simulink model "NumSim_standard_eVTOL"  (R2024b)
settings: Solver=ode14x  StartTime=0.0  StopTime=250  FixedStep=0.005  RelTol=1e-3
values from neighbouring files (symbols this model uses):
  aDl =     [initdata.mat]
  aDr =     [initdata.mat]
  aDyn =     [initdata.mat]
  Airport = init_airport('PHNL')    [initdata_HIL_eVTOL.m]
  aLat =     [initdata.mat]
  aLon =     [initdata.mat]
  D = Prop.D    [EOM_dt_MC.m]    (also in EOM_get_alf_dt_de_prop_evtol.m = CD * QS)
  dt0 = X(2)    [EOM_get_alf_dt_de_prop_evtol.m]    (also in initdata.mat = 0.258252593971; initdata_HIL_eVTOL.m = EOM_dt_MC)
  EAS0 = TAS0 / EAS2TAS    [initdata_HIL_eVTOL.m]
  FCS = init_FCS    [initdata_HIL_eVTOL.m]
  General = init_layoutdata    [EOM_dt_MC.m]    (also in build_optimized_CA.m; initdata.mat = ; initdata_HIL_eVTOL.m)
  h0 = Con(1)    [EOM_get_alf_dt_de_prop_evtol.m]    (also in initdata.mat = 450; initdata_HIL_eVTOL.m = 50)
  mass = Con(3)    [EOM_get_alf_dt_de_prop_evtol.m]    (also in initdata.mat = 2255.54; initdata_HIL_eVTOL.m = 7)
  Motor = init_motor_evtol    [EOM_dt_MC.m]    (also in initdata.mat = []; initdata_HIL_eVTOL.m)
  Prop = init_propeller_evtol_new    [EOM_dt_MC.m]    (also in initdata_HIL_eVTOL.m)
  R2D = 180/pi    (= 57.2957795131)    [EOM_get_alf_dt_de_prop_evtol.m]    (also in init_FCS.m; init_aerodata_evtol.m; init_airport.m; initdata.mat)
  theta0 = -0.0510981441662    [initdata.mat]
undefined symbols (not defined in the file or in its folder): A1, aDa, aDe, asbhl20env, B1, C1, de0, Earth, Environment, InitData, Kd, Kp, magnitude, Tc, WGS84
libraries: simulink_extras x26, simulink x18, slpidlib x14, vrlib x8, matrix_library x6, sharedutil x6, sharedtransform x5, aerolibwindfilters x4, aerolibatmos2 x3, aerolibobsolete x2, aerolibactuator x2, aerolibasang x2
(part 6 of 7)

== system NumSim_standard_eVTOL/Environment/Wind Models/Dryden Wind Turbulence Model (Continuous (+q -r))/Select angular rates/Interpolate rates ==
  pgw_h&l : Inport
  qgw_h&l : Inport  Port=2
  rgw_h&l : Inport  Port=3
  DCM : Inport  Port=4
  Wind direction : Inport  Port=5
  Altitude : Inport  Port=6
  Action Port : ActionPort  PropagateVarSize=During execution  ActionPortLabel=else
  Mux : Mux  Inputs=3
  Mux1 : Mux  Inputs=3
  Product1 : Product  Inputs=**/  SaturateOnIntegerOverflow=on  OutDataTypeStr=Inherit: Same as first input
  Selector : Selector  InputPortWidth=2  IndexOptions=Index vector (dialog)  Indices=1  OutputSizes=1
  Selector1 : Selector  InputPortWidth=2  IndexOptions=Index vector (dialog)  Indices=1  OutputSizes=1
  Selector2 : Selector  InputPortWidth=2  IndexOptions=Index vector (dialog)  Indices=1  OutputSizes=1
  Selector3 : Selector  InputPortWidth=2  IndexOptions=Index vector (dialog)  Indices=2  OutputSizes=1
  Selector4 : Selector  InputPortWidth=2  IndexOptions=Index vector (dialog)  Indices=2  OutputSizes=1
  Selector5 : Selector  InputPortWidth=2  IndexOptions=Index vector (dialog)  Indices=2  OutputSizes=1
  Sum : Sum  Inputs=|-+  SaturateOnIntegerOverflow=on
  Sum1 : Sum  Inputs=|+-  SaturateOnIntegerOverflow=on
  Sum2 : Sum  Inputs=-+|  SaturateOnIntegerOverflow=on
  Sum3 : Sum  Inputs=++|  SaturateOnIntegerOverflow=on
  max_height_low : Constant  Value=max_height_low
  min_height_high : Constant  Value=min_height_high
  wind to body transformation : Subsystem
  pgw,qgw,rgw : Outport  InitialOutput=0  VectorParamsAs1DForOutWhenUnconnected=off
  wires:
  Mux/1 -> wind to body transformation/3(pg_l,qg_l,rg_l)
  DCM/1 -> wind to body transformation/1(DCM)
  wind to body transformation/1(pg,qg,rg) -> Sum3/1, Sum2/1
  Sum3/1 -> pgw,qgw,rgw/1
  Product1/1 -> Sum3/2
  Mux1/1 -> Sum2/2
  Sum2/1 -> Product1/1
  Sum1/1 -> Product1/2
  Sum/1 -> Product1/3
  Altitude/1 -> Sum1/1
  min_height_high/1 -> Sum/2
  max_height_low/1 -> Sum1/2, Sum/1
  Wind direction/1 -> wind to body transformation/2(Wind direction)
  Selector3/1 -> Mux1/1
  Selector4/1 -> Mux1/2
  Selector5/1 -> Mux1/3
  pgw_h&l/1 -> Selector/1, Selector3/1
  qgw_h&l/1 -> Selector4/1, Selector1/1
  rgw_h&l/1 -> Selector5/1, Selector2/1
  Selector/1 -> Mux/1
  Selector1/1 -> Mux/2
  Selector2/1 -> Mux/3

== system NumSim_standard_eVTOL/Environment/Wind Models/Dryden Wind Turbulence Model (Continuous (+q -r))/Select angular rates/Low altitude rates ==
  DCM : Inport
  pgw_h&l : Inport  Port=2
  qgw_h&l : Inport  Port=3
  rgw_h&l : Inport  Port=4
  Wind direction : Inport  Port=5
  Action Port : ActionPort  PropagateVarSize=During execution  ActionPortLabel=if(u1<=max_height_low)
  Mux : Mux  Inputs=3
  Selector : Selector  InputPortWidth=2  IndexOptions=Index vector (dialog)  Indices=1  OutputSizes=1
  Selector1 : Selector  InputPortWidth=2  IndexOptions=Index vector (dialog)  Indices=1  OutputSizes=1
  Selector2 : Selector  InputPortWidth=2  IndexOptions=Index vector (dialog)  Indices=1  OutputSizes=1
  wind to body transformation : Subsystem
  pgw,qgw,rgw : Outport  InitialOutput=0  VectorParamsAs1DForOutWhenUnconnected=off
  wires:
  DCM/1 -> wind to body transformation/1(DCM)
  pgw_h&l/1 -> Selector/1
  qgw_h&l/1 -> Selector1/1
  rgw_h&l/1 -> Selector2/1
  Selector/1 -> Mux/1
  Selector1/1 -> Mux/2
  Selector2/1 -> Mux/3
  Mux/1 -> wind to body transformation/3(pg_l,qg_l,rg_l)
  wind to body transformation/1(pg,qg,rg) -> pgw,qgw,rgw/1
  Wind direction/1 -> wind to body transformation/2(Wind direction)

== system NumSim_standard_eVTOL/Environment/Wind Models/Dryden Wind Turbulence Model (Continuous (+q -r))/Select angular rates/Medium//High altitude rates ==
  pgw_h&l : Inport
  qgw_h&l : Inport  Port=2
  rgw_h&l : Inport  Port=3
  Action Port : ActionPort  PropagateVarSize=During execution  ActionPortLabel=elseif(u1>=min_height_high)
  Gain : Gain  SaturateOnIntegerOverflow=on  OutDataTypeStr=Inherit: Same as input  ParamDataTypeStr=Inherit: Same as input
  Mux : Mux  Inputs=3
  Selector3 : Selector  InputPortWidth=6  IndexOptions=Index vector (dialog)  Indices=[ 2 4 6]  OutputSizes=1
  pgw,qgw,rgw : Outport  InitialOutput=0  VectorParamsAs1DForOutWhenUnconnected=off
  wires:
  Gain/1 -> pgw,qgw,rgw/1
  Selector3/1 -> Gain/1
  pgw_h&l/1 -> Mux/1
  qgw_h&l/1 -> Mux/2
  rgw_h&l/1 -> Mux/3
  Mux/1 -> Selector3/1

== system NumSim_standard_eVTOL/Environment/Wind Models/Dryden Wind Turbulence Model (Continuous (+q -r))/Select angular rates/Merge Subsystems ==
  low : Inport
  high : Inport  Port=2
  interpolated : Inport  Port=3
  Demux : Demux  Outputs=3
      settings: DisplayOption=none
  Merge : Merge  Inputs=3
  pgw : Outport  VectorParamsAs1DForOutWhenUnconnected=off
  qgw : Outport  Port=2  VectorParamsAs1DForOutWhenUnconnected=off
  rgw : Outport  Port=3  VectorParamsAs1DForOutWhenUnconnected=off
  wires:
  low/1 -> Merge/1
  high/1 -> Merge/2
  interpolated/1 -> Merge/3
  Demux/2 -> qgw/1
  Demux/3 -> rgw/1
  Demux/1 -> pgw/1
  Merge/1 -> Demux/1

== system NumSim_standard_eVTOL/Environment/Wind Models/Dryden Wind Turbulence Model (Continuous (+q -r))/Select velocities/Interpolate velocities ==
  ugw_h&l : Inport
  vgw_h&l : Inport  Port=2
  wgw_h&l : Inport  Port=3
  DCM : Inport  Port=4
  Wind direction : Inport  Port=5
  Altitude : Inport  Port=6
  Action Port : ActionPort  PropagateVarSize=During execution  ActionPortLabel=else
  Mux : Mux  Inputs=3
  Mux1 : Mux  Inputs=3
  Product1 : Product  Inputs=**/  SaturateOnIntegerOverflow=on  OutDataTypeStr=Inherit: Same as first input
  Selector : Selector  InputPortWidth=2  IndexOptions=Index vector (dialog)  Indices=1  OutputSizes=1
  Selector1 : Selector  InputPortWidth=2  IndexOptions=Index vector (dialog)  Indices=1  OutputSizes=1
  Selector2 : Selector  InputPortWidth=2  IndexOptions=Index vector (dialog)  Indices=1  OutputSizes=1
  Selector3 : Selector  InputPortWidth=2  IndexOptions=Index vector (dialog)  Indices=2  OutputSizes=1
  Selector4 : Selector  InputPortWidth=2  IndexOptions=Index vector (dialog)  Indices=2  OutputSizes=1
  Selector5 : Selector  InputPortWidth=2  IndexOptions=Index vector (dialog)  Indices=2  OutputSizes=1
  Sum : Sum  Inputs=|-+  SaturateOnIntegerOverflow=on
  Sum1 : Sum  Inputs=|+-  SaturateOnIntegerOverflow=on
  Sum2 : Sum  Inputs=-+|  SaturateOnIntegerOverflow=on
  Sum3 : Sum  Inputs=++|  SaturateOnIntegerOverflow=on
  max_height_low : Constant  Value=max_height_low
  min_height_high : Constant  Value=min_height_high
  wind to body transformation : Subsystem
  ugw,vgw,wgw : Outport  InitialOutput=0  VectorParamsAs1DForOutWhenUnconnected=off
  wires:
  Mux/1 -> wind to body transformation/3(ug_l,vg_l,wg_l)
  Wind direction/1 -> wind to body transformation/2(Wind direction)
  DCM/1 -> wind to body transformation/1(DCM)
  wind to body transformation/1(ug,vg,wg) -> Sum3/1, Sum2/1
  Sum3/1 -> ugw,vgw,wgw/1
  Product1/1 -> Sum3/2
  Mux1/1 -> Sum2/2
  Sum2/1 -> Product1/1
  Sum1/1 -> Product1/2
  Sum/1 -> Product1/3
  Altitude/1 -> Sum1/1
  min_height_high/1 -> Sum/2
  max_height_low/1 -> Sum1/2, Sum/1
  Selector3/1 -> Mux1/1
  Selector4/1 -> Mux1/2
  Selector5/1 -> Mux1/3
  ugw_h&l/1 -> Selector/1, Selector3/1
  vgw_h&l/1 -> Selector4/1, Selector1/1
  wgw_h&l/1 -> Selector5/1, Selector2/1
  Selector/1 -> Mux/1
  Selector1/1 -> Mux/2
  Selector2/1 -> Mux/3

== system NumSim_standard_eVTOL/Environment/Wind Models/Dryden Wind Turbulence Model (Continuous (+q -r))/Select velocities/Low altitude velocities ==
  DCM : Inport
  ugw_h&l : Inport  Port=2
  vgw_h&l : Inport  Port=3
  wgw_h&l : Inport  Port=4
  Wind direction : Inport  Port=5
  Action Port : ActionPort  PropagateVarSize=During execution  ActionPortLabel=if(u1<=max_height_low)
  Mux : Mux  Inputs=3
  Selector : Selector  InputPortWidth=2  IndexOptions=Index vector (dialog)  Indices=1  OutputSizes=1
  Selector1 : Selector  InputPortWidth=2  IndexOptions=Index vector (dialog)  Indices=1  OutputSizes=1
  Selector2 : Selector  InputPortWidth=2  IndexOptions=Index vector (dialog)  Indices=1  OutputSizes=1
  wind to body transformation : Subsystem
  ugw,vgw,wgw : Outport  InitialOutput=0  VectorParamsAs1DForOutWhenUnconnected=off
  wires:
  Mux/1 -> wind to body transformation/3(ug_l,vg_l,wg_l)
  Selector2/1 -> Mux/3
  wind to body transformation/1(ug,vg,wg) -> ugw,vgw,wgw/1
  Wind direction/1 -> wind to body transformation/2(Wind direction)
  DCM/1 -> wind to body transformation/1(DCM)
  Selector1/1 -> Mux/2
  Selector/1 -> Mux/1
  wgw_h&l/1 -> Selector2/1
  vgw_h&l/1 -> Selector1/1
  ugw_h&l/1 -> Selector/1

== system NumSim_standard_eVTOL/Environment/Wind Models/Dryden Wind Turbulence Model (Continuous (+q -r))/Select velocities/Medium//High altitude velocities ==
  ugw_h&l : Inport
  vgw_h&l : Inport  Port=2
  wgw_h&l : Inport  Port=3
  Action Port : ActionPort  PropagateVarSize=During execution  ActionPortLabel=elseif(u1>=min_height_high)
  Gain : Gain  SaturateOnIntegerOverflow=on  OutDataTypeStr=Inherit: Same as input  ParamDataTypeStr=Inherit: Same as input
  Mux : Mux  Inputs=3
  Selector3 : Selector  InputPortWidth=6  IndexOptions=Index vector (dialog)  Indices=[ 2 4 6]  OutputSizes=1
  ugw,vgw,wgw : Outport  InitialOutput=0  VectorParamsAs1DForOutWhenUnconnected=off
  wires:
  vgw_h&l/1 -> Mux/2
  Gain/1 -> ugw,vgw,wgw/1
  Selector3/1 -> Gain/1
  Mux/1 -> Selector3/1
  wgw_h&l/1 -> Mux/3
  ugw_h&l/1 -> Mux/1

== system NumSim_standard_eVTOL/Environment/Wind Models/Dryden Wind Turbulence Model (Continuous (+q -r))/Select velocities/Merge Subsystems ==
  low : Inport
  high : Inport  Port=2
  interpolated : Inport  Port=3
  Demux : Demux  Outputs=3
      settings: DisplayOption=none
  Merge : Merge  Inputs=3
  ugw : Outport  VectorParamsAs1DForOutWhenUnconnected=off
  vgw : Outport  Port=2  VectorParamsAs1DForOutWhenUnconnected=off
  wgw : Outport  Port=3  VectorParamsAs1DForOutWhenUnconnected=off
  wires:
  Merge/1 -> Demux/1
  Demux/1 -> ugw/1
  Demux/3 -> wgw/1
  Demux/2 -> vgw/1
  interpolated/1 -> Merge/3
  high/1 -> Merge/2
  low/1 -> Merge/1

== system NumSim_standard_eVTOL/Environment/Wind Models/Dryden Wind Turbulence Model (Continuous (+q -r))/Turbulence scale lengths/Low altitude scale length ==
  h : Inport
  Limit Function 10ft to 1000ft : Saturate  UpperLimit=max_height_low  LowerLimit=10
  Low Altitude Scale Length : Fcn  Expr=u(1)/(0.177+0.000823*u(1))^1.2
  L_ug L_vg : Outport  InitialOutput=0  VectorParamsAs1DForOutWhenUnconnected=off
  L_wg : Outport  Port=2  InitialOutput=0  VectorParamsAs1DForOutWhenUnconnected=off
  wires:
  h/1 -> Limit Function 10ft to 1000ft/1
  Low Altitude Scale Length/1 -> L_ug L_vg/1
  Limit Function 10ft to 1000ft/1 -> L_wg/1, Low Altitude Scale Length/1

== system NumSim_standard_eVTOL/Environment/Wind Models/Dryden Wind Turbulence Model (Continuous (+q -r))/Turbulence scale lengths/Medium//High altitude scale length ==
  Length Conversion : Subsystem
  Medium/High Altitude : Constant  Value=L_high
  L_ug L_vg L_wg : Outport  Unit=ft  InitialOutput=0  VectorParamsAs1DForOutWhenUnconnected=off
  wires:
  Medium/High Altitude/1 -> Length Conversion/1(in)
  Length Conversion/1(out) -> L_ug L_vg L_wg/1

== system NumSim_standard_eVTOL/FCS/FW/TECS/TECS PX4 & AP201/1st order filter2 ==
  In1 : Inport
  Delay : Delay  DelayLength=1
  Gain : Gain  Gain=0.05
  Gain1 : Gain  Gain=0.95
  Sum : Sum  Inputs=|++
  Out1 : Outport  VectorParamsAs1DForOutWhenUnconnected=off
  wires:
  Sum/1 -> Gain1/1, Out1/1
  Gain/1 -> Sum/1
  Delay/1 -> Sum/2
  Gain1/1 -> Delay/1
  In1/1 -> Gain/1

== system NumSim_standard_eVTOL/FCS/FW/TECS/TECS PX4 & AP201/thetac_AP201 ==
  LonMod : Inport
  SPE_RATE_C : Inport  Port=2
  SKE_RATE_C : Inport  Port=3
  SPE_RATE : Inport  Port=4
  SKE_RATE : Inport  Port=5
  Add15 : Sum  Inputs=+-|
  Add18 : Sum  Inputs=+-|
  Add20 : Sum  Inputs=+-|
  Add3 : Sum  Inputs=++|
  Detect Change : simulink/Logic and Bit Operations/Detect Change  vinit=0  OutDataTypeStr=boolean
  Divide{5..6,11..12} (4 alike) : Product  Inputs=**
  Divide7 : Product  Inputs=*/
  Integrator : Integrator  ExternalReset=either  LimitOutput=on  UpperSaturationLimit=FCS.theta_max*0.6  LowerSaturationLimit=FCS.theta_min*0.6  ZeroCross=off
  KEI : Gain  Gain=0.2
  "KEP " : Gain  Gain=0.2
  Radians to Degrees : simulink_extras/Transformations/Radians to Degrees
  Saturation Dynamic2 : simulink/Discontinuities/Saturation Dynamic  OutMin=[]  OutMax=[]  OutDataTypeStr=Inherit: Same as second input  OutDataType=fixdt(1, 16)  OutScaling=2^-10  DoSatur=off
  dD_dot scp : Scope
  g1 : Gain  Gain=9.8
  thetac scp1 : Scope
  thetac_AP1 : Scope  NumInputPorts=2
  thetac_AP201 : Scope  NumInputPorts=2
  thetac : Outport  VectorParamsAs1DForOutWhenUnconnected=off
  wires:
  [V] -> g1/1
  g1/1 -> Divide7/2
  Divide7/1 -> KEI/1, "KEP "/1, dD_dot scp/1  "dD_dot"
  KEI/1 -> Integrator/1
  SPE_RATE_C/1 -> Divide5/1
  [theta_min] -> Saturation Dynamic2/3
  Divide12/1 -> Add18/2
  [SPE_wt] -> Divide11/2, Divide5/2  "SPE_WT"
  [SKE_wt] -> Divide12/2, Divide6/2  "SKE_WT"
  Add20/1 -> Divide7/1  "SEB_rate_err"
  SKE_RATE/1 -> Divide12/1
  Integrator/1 -> Add3/1, thetac_AP201/1
  [theta_max] -> Saturation Dynamic2/1
  SKE_RATE_C/1 -> Divide6/1
  Divide5/1 -> Add15/1
  Divide6/1 -> Add15/2
  Add15/1 -> Add20/1  "SEB_rate_c"
  SPE_RATE/1 -> Divide11/1
  Add18/1 -> Add20/2  "SEB_rate"
  Divide11/1 -> Add18/1
  "KEP "/1 -> thetac_AP201/2, Add3/2
  Saturation Dynamic2/1 -> Radians to Degrees/1, thetac/1
  Add3/1 -> Saturation Dynamic2/2
  LonMod/1 -> thetac_AP1/1, Detect Change/1
  Detect Change/1 -> thetac_AP1/2, Integrator/2
  Radians to Degrees/1 -> thetac scp1/1

== system NumSim_standard_eVTOL/FCS/FW/TECS/TECS PX4 & AP201/throttlec_AP201 ==
  LonMod : Inport
  SPE_RATE_C : Inport  Port=2
  SKE_RATE_C : Inport  Port=3
  SPE_RATE : Inport  Port=4
  SKE_RATE : Inport  Port=5
  Add2 : Sum  Inputs=++|
  Add6 : Sum  Inputs=++|
  Add7 : Sum  Inputs=++|
  Add9 : Sum  Inputs=+-|
  Detect Change : simulink/Logic and Bit Operations/Detect Change  vinit=0  OutDataTypeStr=boolean
  Divide2 : Product  Inputs=*/
  Integrator1 : Integrator  ExternalReset=either  LimitOutput=on  UpperSaturationLimit=0.5  LowerSaturationLimit=-0.5  ZeroCross=off
  KTI : Gain  Gain=0.8
  KTP : Gain  Gain=0.4
  PX4 1st order filter (time depended)1 : CustomLib/PX4 1st order filter (time depended)  Commented=on  Ts=0.2
  Rate Limiter Dynamic1 : simulink/Discontinuities/Rate Limiter Dynamic
  Saturation Dynamic : simulink/Discontinuities/Saturation Dynamic  OutMin=[]  OutMax=[]  OutDataTypeStr=Inherit: Same as second input  OutDataType=fixdt(1, 16)  OutScaling=2^-10  DoSatur=off
  Saturation3 : Saturate  UpperLimit=1  LowerLimit=-1
  dE_dot scp : Scope
  dt scp{2..5} (4 alike) : Scope
  dt_slew : Constant  Value=0.8
  dti scp1 : Scope  NumInputPorts=2
  g12 : Gain  Gain=9.8
  g13 : Gain  Gain=-1
  dt : Outport  VectorParamsAs1DForOutWhenUnconnected=off
  wires:
  Add2/1 -> Rate Limiter Dynamic1/2  "dt"
  Saturation Dynamic/1 -> dt scp4/1, Add9/1  "STE_rate_c"
  Rate Limiter Dynamic1/1 -> Saturation3/1
  [STE_rate_min] -> Saturation Dynamic/3
  Add7/1 -> dt scp5/1, Saturation Dynamic/2  "STE_rate_c"
  Divide2/1 -> dE_dot scp/1, KTI/1, KTP/1  "dE_dot"
  g12/1 -> Divide2/2
  SPE_RATE/1 -> Add6/1
  Add9/1 -> Divide2/1  "STE_rate_err"
  [V] -> g12/1
  KTI/1 -> Integrator1/1
  SKE_RATE/1 -> Add6/2
  KTP/1 -> Add2/2, dti scp1/2
  Add6/1 -> dt scp3/1, Add9/2  "STE_rate"
  SKE_RATE_C/1 -> Add7/2
  SPE_RATE_C/1 -> Add7/1
  [STE_rate_max] -> Saturation Dynamic/1
  Integrator1/1 -> Add2/1, dti scp1/1
  dt_slew/1 -> Rate Limiter Dynamic1/1, g13/1
  g13/1 -> Rate Limiter Dynamic1/3
  Saturation3/1 -> dt/1, dt scp2/1
  LonMod/1 -> Detect Change/1
  Detect Change/1 -> Integrator1/2

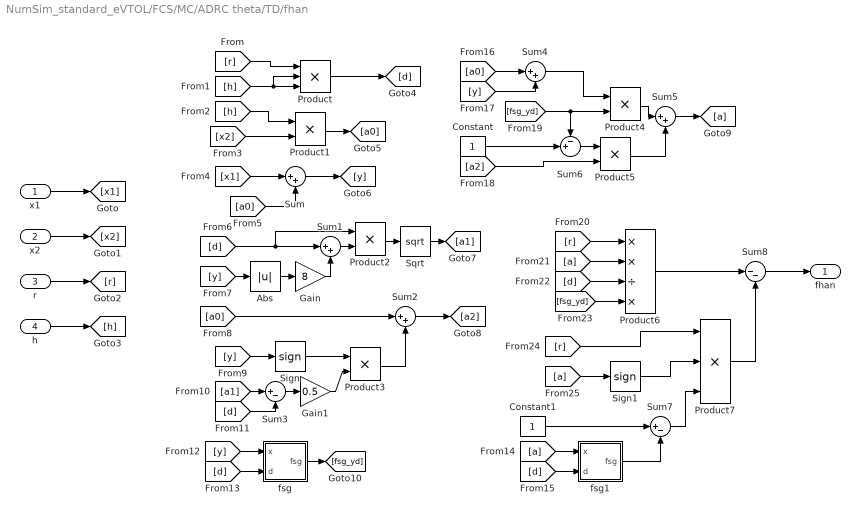
== system NumSim_standard_eVTOL/FCS/MC/ADRC theta/TD/fhan ==
  x1 : Inport
  x2 : Inport  Port=2
  r : Inport  Port=3
  h : Inport  Port=4
  Abs : Abs  SaturateOnIntegerOverflow=off
  Constant : Constant
  Constant1 : Constant
  Gain : Gain  Gain=8
  Gain1 : Gain  Gain=0.5
  Product : Product  Inputs=3
  Product{1..5} (5 alike) : Product
  Product6 : Product  Inputs=**/*
  Product7 : Product  Inputs=***
  Sign : Signum
  Sign1 : Signum
  Sqrt : Sqrt
  Sum{,1..2,4..5} (5 alike) : Sum  Inputs=|++
  Sum3 : Sum  Inputs=|+-
  Sum6 : Sum  Inputs=-+|
  Sum7 : Sum  Inputs=|+-
  Sum8 : Sum  Inputs=|--
  fsg : Subsystem
  fsg1 : Subsystem
  fhan : Outport
  wires:
  Product/1 -> [d]
  x1/1 -> [x1]
  x2/1 -> [x2]
  r/1 -> [r]
  h/1 -> [h]
  [r] -> Product/1
  [h] -> Product/3, Product/2
  [h] -> Product1/1
  [x2] -> Product1/2
  Product1/1 -> [a0]
  [x1] -> Sum/1
  [a0] -> Sum/2
  Sum/1 -> [y]
  [d] -> Sum1/1, Product2/1
  [y] -> Abs/1
  Abs/1 -> Gain/1
  Gain/1 -> Sum1/2
  Sum1/1 -> Product2/2
  Product2/1 -> Sqrt/1
  [a0] -> Sum2/1
  [y] -> Sign/1
  Sign/1 -> Product3/1
  [a1] -> Sum3/1
  [d] -> Sum3/2
  Sum3/1 -> Gain1/1
  Gain1/1 -> Product3/2
  Product3/1 -> Sum2/2
  Sum2/1 -> [a2]
  [y] -> fsg/1(x)
  [d] -> fsg/2(d)
  [d] -> fsg1/2(d)
  [a] -> fsg1/1(x)
  [a0] -> Sum4/1
  [y] -> Sum4/2
  Sum4/1 -> Product4/1
  Product4/1 -> Sum5/1
  [a2] -> Product5/2
  Constant/1 -> Sum6/2
  Sum6/1 -> Product5/1
  Product5/1 -> Sum5/2
  Sum5/1 -> [a]
  fsg/1(fsg) -> [fsg_yd]
  [fsg_yd] -> Sum6/1, Product4/2
  [r] -> Product6/1
  [a] -> Product6/2
  [d] -> Product6/3
  [fsg_yd] -> Product6/4
  Constant1/1 -> Sum7/1
  fsg1/1(fsg) -> Sum7/2
  [a] -> Sign1/1
  [r] -> Product7/1
  Sign1/1 -> Product7/2
  Sum7/1 -> Product7/3
  Product6/1 -> Sum8/1
  Product7/1 -> Sum8/2
  Sum8/1 -> fhan/1
  Sqrt/1 -> [a1]

== system NumSim_standard_eVTOL/airframe/force moment/aero F&M in body axis/Aerodynamic Coefficients/Actuator Increments ==
  Actuators : Inport
  incid : Inport  Port=2
  Aileron : Subsystem
  Bus Selector1 : BusSelector  OutputSignals=dl,dr,da
  Demux : Demux  Outputs=2
  Sum : Sum  Inputs=+++
  Terminator : Terminator
  V_left : Subsystem
  V_right : Subsystem
  cl : Outport  InitialOutput=0  VectorParamsAs1DForOutWhenUnconnected=off
  wires:
  Actuators/1 -> Bus Selector1/1
  Sum/1 -> cl/1
  V_right/1(dr_Coeff) -> Sum/2
  V_left/1(dl_Coeff) -> Sum/1
  Bus Selector1/1 -> V_left/2(dl)  "<dl>"
  Bus Selector1/3 -> Aileron/2(da)  "<da>"
  incid/1 -> Demux/1
  Demux/1 -> Aileron/1(alpha), V_right/1(alpha), V_left/1(alpha)  "alpha"
  Demux/2 -> Terminator/1  "beta"
  Aileron/1(da_Coeff) -> Sum/3
  Bus Selector1/2 -> V_right/2(dr)  "<dr>"

== system NumSim_standard_eVTOL/airframe/force moment/aero F&M in body axis/Aerodynamic Coefficients/Basic Coefficients ==
  Incid : Inport
  mach : Inport  Port=2
  2-D Lookup Table : Lookup_n-D  NumberOfTableDimensions=1  BreakpointsForDimension1=aLon.alpha  BreakpointsForDimension2=aLon.mach  BreakpointsForDimension3=aLon.flap  Table=aLon.CL  InternalRulePriority=Speed  RndMeth=Simplest
  2-D Lookup Table1 : Lookup_n-D  NumberOfTableDimensions=1  BreakpointsForDimension1=aLon.alpha  BreakpointsForDimension2=aLon.mach  BreakpointsForDimension3=aLon.flap  Table=aLon.CD  InternalRulePriority=Speed  RndMeth=Simplest
  2-D Lookup Table2 : Lookup_n-D  NumberOfTableDimensions=1  BreakpointsForDimension1=aLon.alpha  BreakpointsForDimension2=aLon.mach  BreakpointsForDimension3=aLon.flap  Table=aLon.Cm  InternalRulePriority=Speed  RndMeth=Simplest
  2-D Lookup Table3 : Lookup_n-D  BreakpointsForDimension1=aLat.beta  BreakpointsForDimension2=aLat.alpha  BreakpointsForDimension3=aLat.mach  Table=aLat.dCD  InternalRulePriority=Speed  RndMeth=Simplest
      settings: InputPortMap=u0,u1
  2-D Lookup Table4 : Lookup_n-D  BreakpointsForDimension1=aLat.beta  BreakpointsForDimension2=aLat.alpha  BreakpointsForDimension3=aLat.mach  Table=aLat.dCY  InternalRulePriority=Speed  RndMeth=Simplest
      settings: InputPortMap=u0,u1
  2-D Lookup Table5 : Lookup_n-D  BreakpointsForDimension1=aLat.beta  BreakpointsForDimension2=aLat.alpha  BreakpointsForDimension3=aLat.mach  Table=aLat.dCl  InternalRulePriority=Speed  RndMeth=Simplest
      settings: InputPortMap=u0,u1
  2-D Lookup Table6 : Lookup_n-D  BreakpointsForDimension1=aLat.beta  BreakpointsForDimension2=aLat.alpha  BreakpointsForDimension3=aLat.mach  Table=aLat.dCL  InternalRulePriority=Speed  RndMeth=Simplest
      settings: InputPortMap=u0,u1
  2-D Lookup Table7 : Lookup_n-D  BreakpointsForDimension1=aLat.beta  BreakpointsForDimension2=aLat.alpha  BreakpointsForDimension3=aLat.mach  Table=aLat.dCm  InternalRulePriority=Speed  RndMeth=Simplest
      settings: InputPortMap=u0,u1
  2-D Lookup Table8 : Lookup_n-D  BreakpointsForDimension1=aLat.beta  BreakpointsForDimension2=aLat.alpha  BreakpointsForDimension3=aLat.mach  Table=aLat.dCn  InternalRulePriority=Speed  RndMeth=Simplest
      settings: InputPortMap=u0,u1
  Constant : Constant  Value=0
  Constant1 : Constant  Value=0
  Demux : Demux  Outputs=2
  Display : Display
  Display1 : Display
  Gain : Gain
  Mux1 : Mux  Inputs=6
  Mux2 : Mux  Inputs=6
  Saturation : Saturate  UpperLimit=0.1  LowerLimit=0
  Scope{1..5} (5 alike) : Scope
  Sum5 : Sum  Inputs=+++  InputSameDT=on  SaturateOnIntegerOverflow=on  OutDataTypeStr=Inherit: Same as first input
  cl : Outport  InitialOutput=0  VectorParamsAs1DForOutWhenUnconnected=off
  wires:
  Mux1/1 -> Display/1, Sum5/2
  Demux/1 -> Scope5/1, [alpha]  "alpha"
  Demux/2 -> [beta]  "beta"
  2-D Lookup Table1/1 -> Mux1/2, Scope3/1  "CD"
  Constant1/1 -> Mux1/6, Mux1/4, Mux1/3
  2-D Lookup Table4/1 -> Mux2/3  "dCY"
  2-D Lookup Table5/1 -> Mux2/4  "dCl"
  2-D Lookup Table8/1 -> Mux2/6  "dCn"
  Sum5/1 -> cl/1
  Mux2/1 -> Sum5/3, Display1/1
  Incid/1 -> Demux/1
  [alpha] -> 2-D Lookup Table/1, Scope4/1
  2-D Lookup Table/1 -> Scope2/1, Mux1/1  "CL"
  [alpha] -> 2-D Lookup Table1/1
  [alpha] -> 2-D Lookup Table2/1
  2-D Lookup Table2/1 -> Gain/1  "Cm"
  [beta] -> 2-D Lookup Table6/1
  2-D Lookup Table6/1 -> Mux2/1  "dCL"
  [alpha] -> 2-D Lookup Table6/2
  [alpha] -> 2-D Lookup Table3/2
  [beta] -> 2-D Lookup Table3/1
  2-D Lookup Table3/1 -> Mux2/2  "dCD"
  [beta] -> 2-D Lookup Table4/1
  [alpha] -> 2-D Lookup Table4/2
  [alpha] -> 2-D Lookup Table5/2
  [beta] -> 2-D Lookup Table5/1
  [beta] -> 2-D Lookup Table7/1
  [alpha] -> 2-D Lookup Table7/2
  2-D Lookup Table7/1 -> Mux2/5  "dCm"
  [alpha] -> 2-D Lookup Table8/2
  [beta] -> 2-D Lookup Table8/1
  Constant/1 -> Sum5/1
  Saturation/1 -> Scope1/1, [mach]
  mach/1 -> Saturation/1
  Gain/1 -> Mux1/5

== system NumSim_standard_eVTOL/airframe/force moment/aero F&M in body axis/Aerodynamic Coefficients/Body Rate Damping ==
  Incid : Inport
  pqrn : Inport  Port=2
  alphaDot_n : Inport  Port=3
  1-D Lookup Table : Lookup_n-D  NumberOfTableDimensions=1  BreakpointsForDimension1=aDyn.alpha  BreakpointsForDimension2=aDyn.flap  Table=aDyn.CYp  InternalRulePriority=Speed  RndMeth=Simplest
  1-D Lookup Table1 : Lookup_n-D  NumberOfTableDimensions=1  BreakpointsForDimension1=aDyn.alpha  BreakpointsForDimension2=aDyn.flap  Table=aDyn.Clp  InternalRulePriority=Speed  RndMeth=Simplest
  1-D Lookup Table2 : Lookup_n-D  NumberOfTableDimensions=1  BreakpointsForDimension1=aDyn.alpha  BreakpointsForDimension2=aDyn.flap  Table=aDyn.Cnp  InternalRulePriority=Speed  RndMeth=Simplest
  1-D Lookup Table3 : Lookup_n-D  NumberOfTableDimensions=1  BreakpointsForDimension1=aDyn.alpha  BreakpointsForDimension2=aDyn.flap  Table=aDyn.CYr  InternalRulePriority=Speed  RndMeth=Simplest
  1-D Lookup Table4 : Lookup_n-D  NumberOfTableDimensions=1  BreakpointsForDimension1=aDyn.alpha  BreakpointsForDimension2=aDyn.flap  Table=aDyn.Clr  InternalRulePriority=Speed  RndMeth=Simplest
  1-D Lookup Table5 : Lookup_n-D  NumberOfTableDimensions=1  BreakpointsForDimension1=aDyn.alpha  BreakpointsForDimension2=aDyn.flap  Table=aDyn.Cnr  InternalRulePriority=Speed  RndMeth=Simplest
  1-D Lookup Table6 : Lookup_n-D  NumberOfTableDimensions=1  BreakpointsForDimension1=aDyn.alpha  BreakpointsForDimension2=aDyn.flap  Table=aDyn.CLq  InternalRulePriority=Speed  RndMeth=Simplest
  1-D Lookup Table7 : Lookup_n-D  NumberOfTableDimensions=1  BreakpointsForDimension1=aDyn.alpha  BreakpointsForDimension2=aDyn.flap  Table=aDyn.Cmq  InternalRulePriority=Speed  RndMeth=Simplest
  1-D Lookup Table8 : Lookup_n-D  NumberOfTableDimensions=1  BreakpointsForDimension1=aDyn.alpha  BreakpointsForDimension2=aDyn.flap  Table=aDyn.CLAlphaDot  InternalRulePriority=Speed  RndMeth=Simplest
  1-D Lookup Table9 : Lookup_n-D  NumberOfTableDimensions=1  BreakpointsForDimension1=aDyn.alpha  BreakpointsForDimension2=aDyn.flap  Table=aDyn.CmAlphaDot  InternalRulePriority=Speed  RndMeth=Simplest
  Add : Sum  Inputs=++++
  Constant{,6..7,13} (4 alike) : Constant  Value=0
  Demux : Demux  Outputs=3
  Demux1 : Demux  Outputs=2
  Mux{1..4} (4 alike) : Mux  Inputs=6
  Product{4..7} (4 alike) : Product  InputSameDT=on  SaturateOnIntegerOverflow=on  OutDataTypeStr=Inherit: Same as first input
  Terminator : Terminator
  cl : Outport  InitialOutput=0  VectorParamsAs1DForOutWhenUnconnected=off
  wires:
  Add/1 -> cl/1
  1-D Lookup Table/1 -> Mux1/3  "CYp"
  1-D Lookup Table2/1 -> Mux1/6  "Cnp"
  Mux1/1 -> Product4/1
  1-D Lookup Table1/1 -> Mux1/4  "Clp"
  pqrn/1 -> Demux/1
  Demux/1 -> [p]
  Demux/2 -> [q]
  Demux/3 -> [r]
  Constant/1 -> Mux1/1, Mux1/2, Mux1/5
  1-D Lookup Table7/1 -> Mux2/5  "Cmq"
  1-D Lookup Table6/1 -> Mux2/1  "CLq"
  Mux2/1 -> Product5/1
  1-D Lookup Table3/1 -> Mux3/3  "CYr"
  Mux3/1 -> Product6/1
  1-D Lookup Table4/1 -> Mux3/4  "Clr"
  1-D Lookup Table5/1 -> Mux3/6  "Cnr"
  Constant7/1 -> Mux3/2, Mux3/5, Mux3/1
  Constant13/1 -> Mux4/6, Mux4/4, Mux4/3, Mux4/2
  1-D Lookup Table9/1 -> Mux4/5  "CmAlphaDot"
  1-D Lookup Table8/1 -> Mux4/1  "CLAlphaDot"
  Constant6/1 -> Mux2/4, Mux2/6, Mux2/3, Mux2/2
  [p] -> Product4/2
  [q] -> Product5/2
  [r] -> Product6/2
  Mux4/1 -> Product7/1
  alphaDot_n/1 -> Product7/2
  Product4/1 -> Add/1
  Product7/1 -> Add/4
  Demux1/2 -> Terminator/1  "beta"
  Demux1/1 -> [alpha]  "alpha"
  Incid/1 -> Demux1/1
  Product5/1 -> Add/3
  [alpha] -> 1-D Lookup Table3/1, 1-D Lookup Table4/1, 1-D Lookup Table9/1, 1-D Lookup Table8/1, 1-D Lookup Table7/1, 1-D Lookup Table6/1, 1-D Lookup Table5/1, 1-D Lookup Table2/1, 1-D Lookup Table1/1, 1-D Lookup Table/1
  Product6/1 -> Add/2

== system NumSim_standard_eVTOL/airframe/force moment/aero F&M in body axis/Aerodynamic Coefficients/CLCDCY-CXCYCZ ==
  Incid : Inport
  Cl_LDY : Inport  Port=2
  Cl_xA : Fcn  Expr=-u[4]*cos(u[2])*cos(u[1])+u[3]*sin(u[1])
  Cl_yA : Fcn  Expr=-u[4]*sin(u[2])+u[5]
  Cl_zA : Fcn  Expr=-u[4]*cos(u[2])*sin(u[1])-u[3]*cos(u[1])
  Mux : Mux  Inputs=3
  Mux1 : Mux  Inputs=2
  Cl_XYZ : Outport  VectorParamsAs1DForOutWhenUnconnected=off
  wires:
  Mux/1 -> Cl_XYZ/1
  Cl_LDY/1 -> Mux1/2
  Incid/1 -> Mux1/1
  Cl_zA/1 -> Mux/3
  Cl_yA/1 -> Mux/2
  Cl_xA/1 -> Mux/1
  Mux1/1 -> Cl_zA/1, Cl_yA/1, Cl_xA/1

== system NumSim_standard_eVTOL/Environment/Wind Models/Dryden Wind Turbulence Model (Continuous (+q -r))/Select angular rates/Interpolate rates/wind to body transformation ==
  DCM : Inport
  Wind direction : Inport  Port=2
  pg_l,qg_l,rg_l : Inport  Port=3
  Demux : Demux  Outputs=3
      settings: DisplayOption=none
  Product : Product  Multiplication=Matrix(*)  SaturateOnIntegerOverflow=on  OutDataTypeStr=Inherit: Same as first input
  Reshape : Reshape  OutputDimensionality=Customize  OutputDimensions=[3,1]
  Reshape1 : Reshape
  Vector Concatenate : Concatenate  NumInputs=3
  convert to earth coords : Subsystem
  pg,qg,rg : Outport  VectorParamsAs1DForOutWhenUnconnected=off
  wires:
  Reshape1/1 -> pg,qg,rg/1
  Reshape/1 -> Product/2
  DCM/1 -> Product/1
  Wind direction/1 -> convert to earth coords/1(Wind direction)
  convert to earth coords/1(pg) -> Vector Concatenate/1
  convert to earth coords/2(qg) -> Vector Concatenate/2
  Vector Concatenate/1 -> Reshape/1
  Demux/1 -> convert to earth coords/2(pg_l)
  Demux/2 -> convert to earth coords/3(qg_l)
  Demux/3 -> Vector Concatenate/3
  Product/1 -> Reshape1/1
  pg_l,qg_l,rg_l/1 -> Demux/1

== system NumSim_standard_eVTOL/Environment/Wind Models/Dryden Wind Turbulence Model (Continuous (+q -r))/Select angular rates/Low altitude rates/wind to body transformation ==
  DCM : Inport
  Wind direction : Inport  Port=2
  pg_l,qg_l,rg_l : Inport  Port=3
  Demux : Demux  Outputs=3
      settings: DisplayOption=none
  Product : Product  Multiplication=Matrix(*)  SaturateOnIntegerOverflow=on  OutDataTypeStr=Inherit: Same as first input
  Reshape : Reshape  OutputDimensionality=Column vector (2-D)
  Reshape1 : Reshape
  Vector Concatenate : Concatenate  NumInputs=3
  convert to earth coords : Subsystem
  pg,qg,rg : Outport  VectorParamsAs1DForOutWhenUnconnected=off
  wires:
  pg_l,qg_l,rg_l/1 -> Demux/1
  Product/1 -> Reshape1/1
  Demux/3 -> Vector Concatenate/3
  Demux/2 -> convert to earth coords/3(qg_l)
  Demux/1 -> convert to earth coords/2(pg_l)
  Vector Concatenate/1 -> Reshape/1
  convert to earth coords/2(qg) -> Vector Concatenate/2
  convert to earth coords/1(pg) -> Vector Concatenate/1
  Wind direction/1 -> convert to earth coords/1(Wind direction)
  DCM/1 -> Product/1
  Reshape/1 -> Product/2
  Reshape1/1 -> pg,qg,rg/1

== system NumSim_standard_eVTOL/Environment/Wind Models/Dryden Wind Turbulence Model (Continuous (+q -r))/Select velocities/Interpolate velocities/wind to body transformation ==
  DCM : Inport
  Wind direction : Inport  Port=2
  ug_l,vg_l,wg_l : Inport  Port=3
  Demux : Demux  Outputs=3
      settings: DisplayOption=none
  Product : Product  Multiplication=Matrix(*)  SaturateOnIntegerOverflow=on  OutDataTypeStr=Inherit: Same as first input
  Reshape : Reshape  OutputDimensionality=Customize  OutputDimensions=[3,1]
  Reshape1 : Reshape
  Vector Concatenate : Concatenate  NumInputs=3
  convert to earth coords : Subsystem
  ug,vg,wg : Outport  VectorParamsAs1DForOutWhenUnconnected=off
  wires:
  Reshape1/1 -> ug,vg,wg/1
  Reshape/1 -> Product/2
  ug_l,vg_l,wg_l/1 -> Demux/1
  Product/1 -> Reshape1/1
  Demux/3 -> Vector Concatenate/3
  Demux/2 -> convert to earth coords/3(vg_l)
  Demux/1 -> convert to earth coords/2(ug_l)
  Vector Concatenate/1 -> Reshape/1
  convert to earth coords/2(vg) -> Vector Concatenate/2
  convert to earth coords/1(ug) -> Vector Concatenate/1
  Wind direction/1 -> convert to earth coords/1(Wind direction)
  DCM/1 -> Product/1

== system NumSim_standard_eVTOL/Environment/Wind Models/Dryden Wind Turbulence Model (Continuous (+q -r))/Select velocities/Low altitude velocities/wind to body transformation ==
  DCM : Inport
  Wind direction : Inport  Port=2
  ug_l,vg_l,wg_l : Inport  Port=3
  Demux : Demux  Outputs=3
      settings: DisplayOption=none
  Product : Product  Multiplication=Matrix(*)  SaturateOnIntegerOverflow=on  OutDataTypeStr=Inherit: Same as first input
  Reshape : Reshape  OutputDimensionality=Column vector (2-D)
  Reshape1 : Reshape
  Vector Concatenate : Concatenate  NumInputs=3
  convert to earth coords : Subsystem
  ug,vg,wg : Outport  VectorParamsAs1DForOutWhenUnconnected=off
  wires:
  DCM/1 -> Product/1
  Wind direction/1 -> convert to earth coords/1(Wind direction)
  convert to earth coords/1(ug) -> Vector Concatenate/1
  convert to earth coords/2(vg) -> Vector Concatenate/2
  Vector Concatenate/1 -> Reshape/1
  Demux/1 -> convert to earth coords/2(ug_l)
  Demux/2 -> convert to earth coords/3(vg_l)
  Demux/3 -> Vector Concatenate/3
  Product/1 -> Reshape1/1
  ug_l,vg_l,wg_l/1 -> Demux/1
  Reshape/1 -> Product/2
  Reshape1/1 -> ug,vg,wg/1

== system NumSim_standard_eVTOL/Environment/Wind Models/Dryden Wind Turbulence Model (Continuous (+q -r))/Turbulence scale lengths/Medium//High altitude scale length/Length Conversion ==
  in : Inport  Unit=m
  Unit Conversion : UnitConversion
  out : Outport  VectorParamsAs1DForOutWhenUnconnected=off
  wires:
  in/1 -> Unit Conversion/1
  Unit Conversion/1 -> out/1

== system NumSim_standard_eVTOL/FCS/MC/ADRC theta/TD/fhan/fsg ==
  x : Inport
  d : Inport  Port=2
  Gain2 : Gain  Gain=0.5
  Sign1 : Signum
  Sign2 : Signum
  Sum4 : Sum  Inputs=|++
  Sum5 : Sum  Inputs=|+-
  Sum6 : Sum  Inputs=|+-
  fsg : Outport
  wires:
  d/1 -> Sum4/2, Sum5/2
  Sum6/1 -> Gain2/1
  Sign2/1 -> Sum6/2
  x/1 -> Sum5/1, Sum4/1
  Sum4/1 -> Sign1/1
  Sign1/1 -> Sum6/1
  Gain2/1 -> fsg/1
  Sum5/1 -> Sign2/1

== system NumSim_standard_eVTOL/FCS/MC/ADRC theta/TD/fhan/fsg1 ==
  x : Inport
  d : Inport  Port=2
  Gain2 : Gain  Gain=0.5
  Sign1 : Signum
  Sign2 : Signum
  Sum4 : Sum  Inputs=|++
  Sum5 : Sum  Inputs=|+-
  Sum6 : Sum  Inputs=|+-
  fsg : Outport
  wires:
  Sum5/1 -> Sign2/1
  Gain2/1 -> fsg/1
  Sign1/1 -> Sum6/1
  Sum4/1 -> Sign1/1
  x/1 -> Sum4/1, Sum5/1
  Sign2/1 -> Sum6/2
  Sum6/1 -> Gain2/1
  d/1 -> Sum5/2, Sum4/2

== system NumSim_standard_eVTOL/airframe/force moment/aero F&M in body axis/Aerodynamic Coefficients/Actuator Increments/Aileron ==
  alpha : Inport
  da : Inport  Port=2
  2-D Lookup Table3 : Lookup_n-D  NumberOfTableDimensions=1  BreakpointsForDimension1=aDa.alpha  BreakpointsForDimension2=aDe.alpha  BreakpointsForDimension3=aDe.flap  Table=aDa.CYDa  InternalRulePriority=Speed  RndMeth=Simplest
  2-D Lookup Table4 : Lookup_n-D  NumberOfTableDimensions=1  BreakpointsForDimension1=aDa.alpha  BreakpointsForDimension2=aDe.alpha  BreakpointsForDimension3=aDe.flap  Table=aDa.ClDa  InternalRulePriority=Speed  RndMeth=Simplest
  2-D Lookup Table5 : Lookup_n-D  NumberOfTableDimensions=1  BreakpointsForDimension1=aDa.alpha  BreakpointsForDimension2=aDe.alpha  BreakpointsForDimension3=aDe.flap  Table=aDa.CnDa  InternalRulePriority=Speed  RndMeth=Simplest
  Constant : Constant  Value=0
  Divide2 : Product  Inputs=**
  Divide3 : Product  Inputs=**
  Divide5 : Product  Inputs=**
  Mux1 : Mux  Inputs=6
  da_Coeff : Outport  VectorParamsAs1DForOutWhenUnconnected=off
  wires:
  alpha/1 -> 2-D Lookup Table5/1, 2-D Lookup Table4/1, 2-D Lookup Table3/1
  Mux1/1 -> da_Coeff/1
  da/1 -> Divide5/1, Divide3/1, Divide2/1
  Divide2/1 -> Mux1/3
  Divide3/1 -> Mux1/4
  2-D Lookup Table3/1 -> Divide2/2
  Divide5/1 -> Mux1/6
  2-D Lookup Table5/1 -> Divide5/2
  2-D Lookup Table4/1 -> Divide3/2
  Constant/1 -> Mux1/5, Mux1/2, Mux1/1

== system NumSim_standard_eVTOL/airframe/force moment/aero F&M in body axis/Aerodynamic Coefficients/Actuator Increments/V_left ==
  alpha : Inport
  dl : Inport  Port=2
  2-D Lookup Table : Lookup_n-D  NumberOfTableDimensions=1  BreakpointsForDimension1=aDl.alpha  BreakpointsForDimension2=aDl.alpha  BreakpointsForDimension3=aDe.flap  Table=aDl.CLDl  InternalRulePriority=Speed  RndMeth=Simplest
  2-D Lookup Table1 : Lookup_n-D  NumberOfTableDimensions=1  BreakpointsForDimension1=aDl.alpha  BreakpointsForDimension2=aDe.alpha  BreakpointsForDimension3=aDe.flap  Table=aDl.CmDl  InternalRulePriority=Speed  RndMeth=Simplest
  2-D Lookup Table2 : Lookup_n-D  NumberOfTableDimensions=1  BreakpointsForDimension1=aDl.alpha  BreakpointsForDimension2=aDe.alpha  BreakpointsForDimension3=aDe.flap  Table=aDl.CDDl  InternalRulePriority=Speed  RndMeth=Simplest
  2-D Lookup Table3 : Lookup_n-D  NumberOfTableDimensions=1  BreakpointsForDimension1=aDl.alpha  BreakpointsForDimension2=aDe.alpha  BreakpointsForDimension3=aDe.flap  Table=aDl.CYDl  InternalRulePriority=Speed  RndMeth=Simplest
  2-D Lookup Table4 : Lookup_n-D  NumberOfTableDimensions=1  BreakpointsForDimension1=aDl.alpha  BreakpointsForDimension2=aDe.alpha  BreakpointsForDimension3=aDe.flap  Table=aDl.ClDl  InternalRulePriority=Speed  RndMeth=Simplest
  2-D Lookup Table5 : Lookup_n-D  NumberOfTableDimensions=1  BreakpointsForDimension1=aDl.alpha  BreakpointsForDimension2=aDe.alpha  BreakpointsForDimension3=aDe.flap  Table=aDl.CnDl  InternalRulePriority=Speed  RndMeth=Simplest
  Divide{,1..5} (6 alike) : Product  Inputs=**
  Mux1 : Mux  Inputs=6
  dl_Coeff : Outport  VectorParamsAs1DForOutWhenUnconnected=off
  wires:
  2-D Lookup Table/1 -> Divide/2
  2-D Lookup Table2/1 -> Divide1/2
  2-D Lookup Table1/1 -> Divide4/2
  Mux1/1 -> dl_Coeff/1
  Divide4/1 -> Mux1/5
  Divide/1 -> Mux1/1
  Divide1/1 -> Mux1/2
  Divide2/1 -> Mux1/3
  2-D Lookup Table3/1 -> Divide2/2
  Divide3/1 -> Mux1/4
  2-D Lookup Table4/1 -> Divide3/2
  dl/1 -> Divide5/1, Divide4/1, Divide3/1, Divide2/1, Divide1/1, Divide/1
  alpha/1 -> 2-D Lookup Table5/1, 2-D Lookup Table1/1, 2-D Lookup Table4/1, 2-D Lookup Table3/1, 2-D Lookup Table2/1, 2-D Lookup Table/1
  2-D Lookup Table5/1 -> Divide5/2
  Divide5/1 -> Mux1/6

== system NumSim_standard_eVTOL/airframe/force moment/aero F&M in body axis/Aerodynamic Coefficients/Actuator Increments/V_right ==
  alpha : Inport
  dr : Inport  Port=2
  2-D Lookup Table : Lookup_n-D  NumberOfTableDimensions=1  BreakpointsForDimension1=aDr.alpha  BreakpointsForDimension2=aDl.alpha  BreakpointsForDimension3=aDe.flap  Table=aDr.CLDr  InternalRulePriority=Speed  RndMeth=Simplest
  2-D Lookup Table1 : Lookup_n-D  NumberOfTableDimensions=1  BreakpointsForDimension1=aDr.alpha  BreakpointsForDimension2=aDe.alpha  BreakpointsForDimension3=aDe.flap  Table=aDr.CmDr  InternalRulePriority=Speed  RndMeth=Simplest
  2-D Lookup Table2 : Lookup_n-D  NumberOfTableDimensions=1  BreakpointsForDimension1=aDr.alpha  BreakpointsForDimension2=aDe.alpha  BreakpointsForDimension3=aDe.flap  Table=aDr.CDDr  InternalRulePriority=Speed  RndMeth=Simplest
  2-D Lookup Table3 : Lookup_n-D  NumberOfTableDimensions=1  BreakpointsForDimension1=aDr.alpha  BreakpointsForDimension2=aDe.alpha  BreakpointsForDimension3=aDe.flap  Table=aDr.CYDr  InternalRulePriority=Speed  RndMeth=Simplest
  2-D Lookup Table4 : Lookup_n-D  NumberOfTableDimensions=1  BreakpointsForDimension1=aDr.alpha  BreakpointsForDimension2=aDe.alpha  BreakpointsForDimension3=aDe.flap  Table=aDr.ClDr  InternalRulePriority=Speed  RndMeth=Simplest
  2-D Lookup Table5 : Lookup_n-D  NumberOfTableDimensions=1  BreakpointsForDimension1=aDr.alpha  BreakpointsForDimension2=aDe.alpha  BreakpointsForDimension3=aDe.flap  Table=aDr.CnDr  InternalRulePriority=Speed  RndMeth=Simplest
  Divide{,1..5} (6 alike) : Product  Inputs=**
  Mux1 : Mux  Inputs=6
  dr_Coeff : Outport  VectorParamsAs1DForOutWhenUnconnected=off
  wires:
  dr/1 -> Divide5/1, Divide4/1, Divide3/1, Divide2/1, Divide1/1, Divide/1
  alpha/1 -> 2-D Lookup Table5/1, 2-D Lookup Table1/1, 2-D Lookup Table4/1, 2-D Lookup Table3/1, 2-D Lookup Table2/1, 2-D Lookup Table/1
  Divide/1 -> Mux1/1
  2-D Lookup Table5/1 -> Divide5/2
  Divide5/1 -> Mux1/6
  2-D Lookup Table1/1 -> Divide4/2
  Divide4/1 -> Mux1/5
  Divide2/1 -> Mux1/3
  2-D Lookup Table4/1 -> Divide3/2
  2-D Lookup Table/1 -> Divide/2
  2-D Lookup Table3/1 -> Divide2/2
  Mux1/1 -> dr_Coeff/1
  Divide3/1 -> Mux1/4
  2-D Lookup Table2/1 -> Divide1/2
  Divide1/1 -> Mux1/2

== system NumSim_standard_eVTOL/Environment/Wind Models/Dryden Wind Turbulence Model (Continuous (+q -r))/Select angular rates/Interpolate rates/wind to body transformation/convert to earth coords ==
  Wind direction : Inport
  pg_l : Inport  Port=2
  qg_l : Inport  Port=3
  Demux : Demux  Outputs=2
      settings: DisplayOption=none
  Demux1 : Demux  Outputs=2
      settings: DisplayOption=none
  Mux : Mux  Inputs=2
  Mux1 : Mux  Inputs=2
  Product1 : Product  InputSameDT=on  SaturateOnIntegerOverflow=on  OutDataTypeStr=Inherit: Same as first input
  Product2 : Product  InputSameDT=on  SaturateOnIntegerOverflow=on  OutDataTypeStr=Inherit: Same as first input
  Selector : Selector  InputPortWidth=4  IndexOptions=Index vector (dialog)  Indices=[1 4]  OutputSizes=1
  Selector1 : Selector  InputPortWidth=4  IndexOptions=Index vector (dialog)  Indices=[2 3]  OutputSizes=1
  Sum : Sum  Inputs=|+-  SaturateOnIntegerOverflow=on
  Sum1 : Sum  Inputs=|++  SaturateOnIntegerOverflow=on
  Trigonometric Function : Trigonometry  Operator=sincos
  pg : Outport  VectorParamsAs1DForOutWhenUnconnected=off
  qg : Outport  Port=2  VectorParamsAs1DForOutWhenUnconnected=off
  wires:
  Trigonometric Function/1 -> Product1/1
  Trigonometric Function/2 -> Product2/2
  Selector1/1 -> Demux1/1
  Selector/1 -> Demux/1
  Mux1/1 -> Selector1/1, Selector/1
  Product1/1 -> Mux1/2
  Product2/1 -> Mux1/1
  Demux1/2 -> Sum1/2
  Demux1/1 -> Sum1/1
  Demux/2 -> Sum/2
  Demux/1 -> Sum/1
  Sum1/1 -> qg/1
  Sum/1 -> pg/1
  Mux/1 -> Product2/1, Product1/2
  qg_l/1 -> Mux/2
  pg_l/1 -> Mux/1
  Wind direction/1 -> Trigonometric Function/1

== system NumSim_standard_eVTOL/Environment/Wind Models/Dryden Wind Turbulence Model (Continuous (+q -r))/Select angular rates/Low altitude rates/wind to body transformation/convert to earth coords ==
  Wind direction : Inport
  pg_l : Inport  Port=2
  qg_l : Inport  Port=3
  Demux : Demux  Outputs=2
      settings: DisplayOption=none
  Demux1 : Demux  Outputs=2
      settings: DisplayOption=none
  Mux : Mux  Inputs=2
  Mux1 : Mux  Inputs=2
  Product1 : Product  InputSameDT=on  SaturateOnIntegerOverflow=on  OutDataTypeStr=Inherit: Same as first input
  Product2 : Product  InputSameDT=on  SaturateOnIntegerOverflow=on  OutDataTypeStr=Inherit: Same as first input
  Selector : Selector  InputPortWidth=4  IndexOptions=Index vector (dialog)  Indices=[1 4]  OutputSizes=1
  Selector1 : Selector  InputPortWidth=4  IndexOptions=Index vector (dialog)  Indices=[2 3]  OutputSizes=1
  Sum : Sum  Inputs=|+-  SaturateOnIntegerOverflow=on
  Sum1 : Sum  Inputs=|++  SaturateOnIntegerOverflow=on
  Trigonometric Function1 : Trigonometry  Operator=sincos
  pg : Outport  VectorParamsAs1DForOutWhenUnconnected=off
  qg : Outport  Port=2  VectorParamsAs1DForOutWhenUnconnected=off
  wires:
  Trigonometric Function1/2 -> Product2/2
  Wind direction/1 -> Trigonometric Function1/1
  pg_l/1 -> Mux/1
  qg_l/1 -> Mux/2
  Trigonometric Function1/1 -> Product1/1
  Mux/1 -> Product1/2, Product2/1
  Sum/1 -> pg/1
  Sum1/1 -> qg/1
  Demux/1 -> Sum/1
  Demux/2 -> Sum/2
  Demux1/1 -> Sum1/1
  Demux1/2 -> Sum1/2
  Product2/1 -> Mux1/1
  Product1/1 -> Mux1/2
  Mux1/1 -> Selector/1, Selector1/1
  Selector/1 -> Demux/1
  Selector1/1 -> Demux1/1

== system NumSim_standard_eVTOL/Environment/Wind Models/Dryden Wind Turbulence Model (Continuous (+q -r))/Select velocities/Interpolate velocities/wind to body transformation/convert to earth coords ==
  Wind direction : Inport
  ug_l : Inport  Port=2
  vg_l : Inport  Port=3
  Demux : Demux  Outputs=2
      settings: DisplayOption=none
  Demux1 : Demux  Outputs=2
      settings: DisplayOption=none
  Mux : Mux  Inputs=2
  Mux1 : Mux  Inputs=2
  Product1 : Product  InputSameDT=on  SaturateOnIntegerOverflow=on  OutDataTypeStr=Inherit: Same as first input
  Product2 : Product  InputSameDT=on  SaturateOnIntegerOverflow=on  OutDataTypeStr=Inherit: Same as first input
  Selector : Selector  InputPortWidth=4  IndexOptions=Index vector (dialog)  Indices=[1 4]  OutputSizes=1
  Selector1 : Selector  InputPortWidth=4  IndexOptions=Index vector (dialog)  Indices=[2 3]  OutputSizes=1
  Sum : Sum  Inputs=|+-  SaturateOnIntegerOverflow=on
  Sum1 : Sum  Inputs=|++  SaturateOnIntegerOverflow=on
  Trigonometric Function : Trigonometry  Operator=sincos
  ug : Outport  VectorParamsAs1DForOutWhenUnconnected=off
  vg : Outport  Port=2  VectorParamsAs1DForOutWhenUnconnected=off
  wires:
  Trigonometric Function/2 -> Product2/2
  Wind direction/1 -> Trigonometric Function/1
  ug_l/1 -> Mux/1
  vg_l/1 -> Mux/2
  Trigonometric Function/1 -> Product1/1
  Mux/1 -> Product1/2, Product2/1
  Sum/1 -> ug/1
  Sum1/1 -> vg/1
  Demux/1 -> Sum/1
  Demux/2 -> Sum/2
  Demux1/1 -> Sum1/1
  Demux1/2 -> Sum1/2
  Product2/1 -> Mux1/1
  Product1/1 -> Mux1/2
  Mux1/1 -> Selector/1, Selector1/1
  Selector/1 -> Demux/1
  Selector1/1 -> Demux1/1

== system NumSim_standard_eVTOL/Environment/Wind Models/Dryden Wind Turbulence Model (Continuous (+q -r))/Select velocities/Low altitude velocities/wind to body transformation/convert to earth coords ==
  Wind direction : Inport
  ug_l : Inport  Port=2
  vg_l : Inport  Port=3
  Demux : Demux  Outputs=2
      settings: DisplayOption=none
  Demux1 : Demux  Outputs=2
      settings: DisplayOption=none
  Mux : Mux  Inputs=2
  Mux1 : Mux  Inputs=2
  Product1 : Product  InputSameDT=on  SaturateOnIntegerOverflow=on  OutDataTypeStr=Inherit: Same as first input
  Product2 : Product  InputSameDT=on  SaturateOnIntegerOverflow=on  OutDataTypeStr=Inherit: Same as first input
  Selector : Selector  InputPortWidth=4  IndexOptions=Index vector (dialog)  Indices=[1 4]  OutputSizes=1
  Selector1 : Selector  InputPortWidth=4  IndexOptions=Index vector (dialog)  Indices=[2 3]  OutputSizes=1
  Sum : Sum  Inputs=|+-  SaturateOnIntegerOverflow=on
  Sum1 : Sum  Inputs=|++  SaturateOnIntegerOverflow=on
  Trigonometric Function : Trigonometry  Operator=sincos
  ug : Outport  VectorParamsAs1DForOutWhenUnconnected=off
  vg : Outport  Port=2  VectorParamsAs1DForOutWhenUnconnected=off
  wires:
  Trigonometric Function/2 -> Product2/2
  Selector1/1 -> Demux1/1
  Selector/1 -> Demux/1
  Mux1/1 -> Selector1/1, Selector/1
  Product1/1 -> Mux1/2
  Product2/1 -> Mux1/1
  Demux1/2 -> Sum1/2
  Demux1/1 -> Sum1/1
  Demux/2 -> Sum/2
  Demux/1 -> Sum/1
  Sum1/1 -> vg/1
  Sum/1 -> ug/1
  Mux/1 -> Product2/1, Product1/2
  Trigonometric Function/1 -> Product1/1
  vg_l/1 -> Mux/2
  ug_l/1 -> Mux/1
  Wind direction/1 -> Trigonometric Function/1

== matlab function NumSim_standard_eVTOL/FCS/MC/Control Allocation ==
  data: da_MC input; dt output; de_MC input; dr_MC input; dt_MC input; pos_plr input; i input
function dt = CA(da_MC, de_MC, dr_MC, dt_MC, pos_plr, i)
    
    L1_x = pos_plr(1);  L1_y = pos_plr(2);
    L2_x = pos_plr(4);  L2_y = pos_plr(5);
    L3_x = pos_plr(7);  L3_y = pos_plr(8);
    L4_x = pos_plr(10); L4_y = pos_plr(11);
    L5_x = pos_plr(13); L5_y = pos_plr(14);
    L6_x = pos_plr(16); L6_y = pos_plr(17);
    
    positions_x = [L1_x, L2_x, L3_x, L4_x, L5_x, L6_x];
    positions_y = [L1_y, L2_y, L3_y, L4_y, L5_y, L6_y];
    max_position = max([abs(positions_x), abs(positions_y)]);

    eff_i = max(i, 0.1); 
    sin_i = sin(eff_i);
    cos_i = cos(eff_i);

    C_thrust = [1/0.509, 1/0.505, 1/0.501, 1/0.501, 1/0.505, 1/0.509]; 
    C_roll   = -positions_y / max_position;                    
    C_pitch  = positions_x / max_position;                     
    C_yaw_Q  = [-1, 1, 1, -1, -1, 1]; 

    CA_dyn = zeros(4, 6);
    CA_dyn(1, :) = C_thrust; 
    CA_dyn(2, :) = C_roll * sin_i;
    CA_dyn(3, :) = C_pitch * sin_i;
    
    K_diff = 1.0; 
    CA_dyn(4, :) = (C_yaw_Q * sin_i) + (C_roll * cos_i * K_diff);

    CA_pinv = pinv(CA_dyn);
    act_MC = [dt_MC; da_MC; de_MC; dr_MC];
    dt0 = CA_pinv * act_MC;

    dt = zeros(6,1);
    for k = 1:6
        dt(k,1) = dt0(k);
    end
end




% function dt = CA(da_MC,de_MC,dr_MC,dt_MC, pos_plr)
% 
% L1_x = pos_plr(1);          
% L1_y = pos_plr(2);
% L2_x = pos_plr(4);
% L2_y = pos_plr(5);
% L3_x = pos_plr(7);
% L3_y = pos_plr(8);
% L4_x = pos_plr(10);
% L4_y = pos_plr(11);
% L5_x = pos_plr(13);
% L5_y = pos_plr(14);
% L6_x = pos_plr(16);
% L6_y = pos_plr(17);
% 
% positions_x = [L1_x, L2_x, L3_x, L4_x, L5_x, L6_x];
% positions_y = [L1_y, L2_y, L3_y, L4_y, L5_y, L6_y];
% 
% max_position = max([abs(positions_x), abs(positions_y)]);
% 
% 
% %thr_MC = zeros(6,1);
% dt = zeros(6,1);
% 
% act_MC = [dt_MC,da_MC,de_MC,dr_MC]';
% 
% CA = [
% 1/0.7   1/0.67 1/0.63 1/0.63 1/0.67 1/0.7  ;
%  -positions_y / max_position; 
%   positions_x / max_position; 
% -1      1      1     -1     -1      1 ];
% 
% CA_pinv = pinv(CA);        %求伪逆
% 
% dt0 = CA_pinv * act_MC;
% 
% dt(1,1) = dt0(1);
% dt(2,1) = dt0(2);
% dt(3,1) = dt0(3);
% dt(4,1) = dt0(4);
% dt(5,1) = dt0(5);
% dt(6,1) = dt0(6);

% thr_MC(1,1) = act_MC * [1, -1, -1, 1]';
% thr_MC(2,1) = act_MC * [-1, 1, -1, 1]';
% thr_MC(3,1) = act_MC * [-1, -1, 1, 1]';
% thr_MC(4,1) = act_MC * [1, 1, 1, 1]';
% thr_MC(5,1) = act_MC * [0, 1, 1]';
% thr_MC(6,1) = act_MC * [1, 1, 1]';

% y = u;

% 控制分配的关系
% [Mx, My, Mz]' = [-0.707, 0, 1] * da
% [Mx, My, Mz]' = [0, 0.707, 0] * de
% [Mx, My, Mz]' = [0, 0, -1] * dr
% 所以只有俯仰偏航时没有操纵耦合，而有滚转控制时应加入dr抵消掉伴生的偏航力矩
% 即如果有da_MC，应交联控制tilt_MC

== stateflow chart NumSim_standard_eVTOL/FCS/FW/V hold//control/dt Fade at 0.1 // sec/Chart ==
  state Flare_dt
    entry:
    dt=dt_ini
  (default) -> Flare_dt
  data: dt_ini input; dt output
